simulink model "BloquesLinealizacionRealimentacionNLDesacoplamiento"  (R2023b)
settings: Solver=VariableStepAuto  StartTime=0.0  StopTime=10.0  RelTol=1e-3
values from neighbouring files (symbols this model uses):
  alfa_cu = 3.9E-3    (= 0.0039)    [Parametros.m]
  b_eq = b_m + b_l/(r^2)    (= 2.19444444444e-05)    [Parametros.m]
  C_ts = 0.818    [Parametros.m]
  g = 9.80665    [Parametros.m]
  J_eq = J_m + J_l/(r^2)    [Parametros.m]
  k_l = m*l_cm + m_l(1)*l_l    [Parametros.m]
  L_d = 6.6E-3    (= 0.0066)    [Parametros.m]
  L_ls = 0.8E-3    (= 0.0008)    [Parametros.m]
  L_q = 5.8E-3    (= 0.0058)    [Parametros.m]
  lambda_m = 0.016    [Parametros.m]
  P_p = 3    [Parametros.m]
  r = 120    [Parametros.m]
  R_tsamb = 146.7    [Parametros.m]
  Rs = 1.02    [Parametros.m]
  Tsref = 20    [Parametros.m]
settings Model: Creator=Home  LastModifiedBy=Home

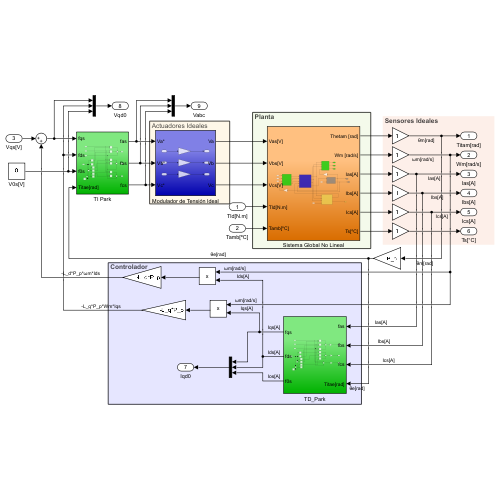
[thumbnail: Simulink's stored preview of the top-level diagram]
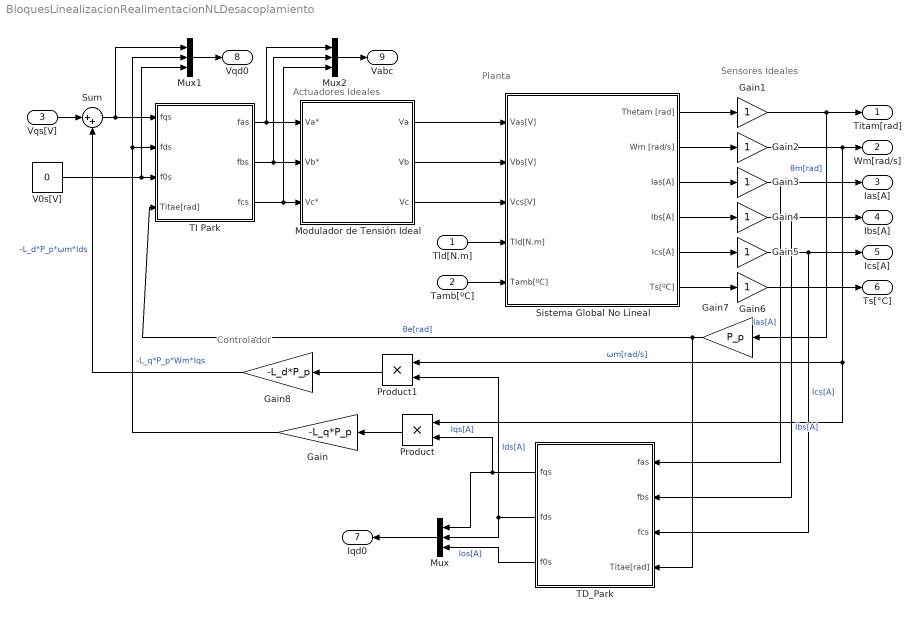
== system BloquesLinealizacionRealimentacionNLDesacoplamiento ==
  note: Planta
  note: Actuadores Ideales
  note: Controlador
  note: Sensores Ideales
  Tld[N.m] : Inport
  Tamb[ºC] : Inport  Port=2
  Vqs[V] : Inport  Port=3
  Gain : Gain  Gain=-L_q*P_p
  Gain{1..6} (6 alike) : Gain
  Gain7 : Gain  Gain=P_p
  Gain8 : Gain  Gain=-L_d*P_p
  Modulador de Tensión Ideal : Subsystem
  Mux : Mux  Inputs=3
  Mux1 : Mux  Inputs=3
  Mux2 : Mux  Inputs=3
  Product : Product
  Product1 : Product
  Sistema Global No Lineal : Subsystem
  Sum : Sum  Inputs=|++
  TD_Park : Subsystem
  TI Park : Subsystem
  V0s[V] : Constant  Value=0
  Titam[rad] : Outport
  Wm[rad/s] : Outport  Port=2
  Ias[A] : Outport  Port=3
  Ibs[A] : Outport  Port=4
  Ics[A] : Outport  Port=5
  Ts[°C] : Outport  Port=6
  Iqd0 : Outport  Port=7
  Vqd0 : Outport  Port=8
  Vabc : Outport  Port=9
  wires:
  Mux2/1 -> Vabc/1
  Sistema Global No Lineal/3(Ias[A]) -> Gain3/1
  Gain5/1 -> TD_Park/3(fcs), Ics[A]/1  "Ics[A]"
  Sistema Global No Lineal/4(Ibs[A]) -> Gain4/1
  Gain2/1 -> Product/1, Product1/1, Wm[rad/s]/1  "ωm[rad/s]"
  TD_Park/1(fqs) -> Mux/1, Product/2  "Iqs[A]"
  Product/1 -> Gain/1
  Tld[N.m]/1 -> Sistema Global No Lineal/4(Tld[N.m])
  TD_Park/2(fds) -> Product1/2, Mux/2  "Ids[A]"
  Gain6/1 -> Ts[°C]/1
  Gain4/1 -> Ibs[A]/1, TD_Park/2(fbs)  "Ibs[A]"
  TI Park/3(fcs) -> Mux2/3, Modulador de Tensión Ideal/3(Vc*)
  Gain3/1 -> TD_Park/1(fas), Ias[A]/1  "Ias[A]"
  Gain/1 -> Mux1/2, TI Park/2(fds)  "-L_q*P_p*Wm*Iqs"
  V0s[V]/1 -> Mux1/3, TI Park/3(f0s)
  Gain7/1 -> TI Park/4(Titae[rad]), TD_Park/4(Titae[rad])  "θe[rad]"
  Sistema Global No Lineal/6(Ts[ºC]) -> Gain6/1
  Sistema Global No Lineal/5(Ics[A]) -> Gain5/1
  Mux/1 -> Iqd0/1
  Modulador de Tensión Ideal/3(Vc) -> Sistema Global No Lineal/3(Vcs[V])
  Sistema Global No Lineal/2(Wm [rad/s]) -> Gain2/1
  Modulador de Tensión Ideal/2(Vb) -> Sistema Global No Lineal/2(Vbs[V])
  Gain1/1 -> Gain7/1, Titam[rad]/1  "θm[rad]"
  TD_Park/3(f0s) -> Mux/3  "Ios[A]"
  Tamb[ºC]/1 -> Sistema Global No Lineal/5(Tamb[ºC])
  TI Park/1(fas) -> Mux2/1, Modulador de Tensión Ideal/1(Va*)
  Sistema Global No Lineal/1(Thetam [rad]) -> Gain1/1
  Modulador de Tensión Ideal/1(Va) -> Sistema Global No Lineal/1(Vas[V])
  TI Park/2(fbs) -> Mux2/2, Modulador de Tensión Ideal/2("Vb* ")
  Mux1/1 -> Vqd0/1
  Product1/1 -> Gain8/1
  Vqs[V]/1 -> Sum/1
  Sum/1 -> Mux1/1, TI Park/1(fqs)
  Gain8/1 -> Sum/2  "-L_d*P_p*ωm*Ids"

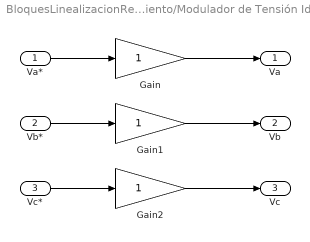
== system BloquesLinealizacionRealimentacionNLDesacoplamiento/Modulador de Tensión Ideal ==
  Va* : Inport
  "Vb* " : Inport  Port=2
  Vc* : Inport  Port=3
  Gain : Gain
  Gain1 : Gain
  Gain2 : Gain
  Va : Outport
  Vb : Outport  Port=2
  Vc : Outport  Port=3
  wires:
  Vc*/1 -> Gain2/1
  "Vb* "/1 -> Gain1/1
  Gain/1 -> Va/1
  Va*/1 -> Gain/1
  Gain1/1 -> Vb/1
  Gain2/1 -> Vc/1

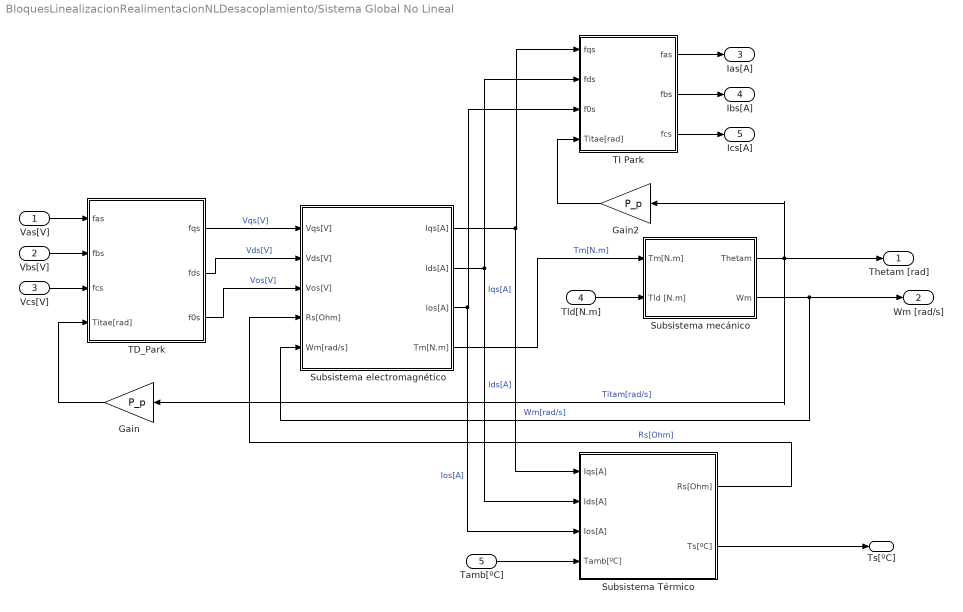
== system BloquesLinealizacionRealimentacionNLDesacoplamiento/Sistema Global No Lineal ==
  Vas[V] : Inport
  Vbs[V] : Inport  Port=2
  Vcs[V] : Inport  Port=3
  Tld[N.m] : Inport  Port=4
  Tamb[ºC] : Inport  Port=5
  Gain : Gain  Gain=P_p
  Gain2 : Gain  Gain=P_p
  Subsistema Térmico : Subsystem
  Subsistema electromagnético : Subsystem
  Subsistema mecánico : Subsystem
  TD_Park : Subsystem
  TI Park : Subsystem
  Thetam [rad] : Outport
  Wm [rad/s] : Outport  Port=2
  Ias[A] : Outport  Port=3
  Ibs[A] : Outport  Port=4
  Ics[A] : Outport  Port=5
  Ts[ºC] : Outport  Port=6
  wires:
  Subsistema electromagnético/3(Ios[A]) -> Subsistema Térmico/3(Ios[A]), TI Park/3(f0s)  "Ios[A]"
  Subsistema mecánico/2(Wm) -> Wm [rad/s]/1, Subsistema electromagnético/5(Wm[rad/s])  "Wm[rad/s]"
  TD_Park/3(f0s) -> Subsistema electromagnético/3(Vos[V])  "Vos[V]"
  Gain/1 -> TD_Park/4(Titae[rad])
  Subsistema Térmico/1(Rs[Ohm]) -> Subsistema electromagnético/4(Rs[Ohm])  "Rs[Ohm]"
  TD_Park/1(fqs) -> Subsistema electromagnético/1(Vqs[V])  "Vqs[V]"
  Vbs[V]/1 -> TD_Park/2(fbs)
  Vcs[V]/1 -> TD_Park/3(fcs)
  Subsistema electromagnético/1(Iqs[A]) -> Subsistema Térmico/1(Iqs[A]), TI Park/1(fqs)  "Iqs[A]"
  Subsistema electromagnético/4(Tm[N.m]) -> Subsistema mecánico/1(Tm[N.m])  "Tm[N.m]"
  Subsistema mecánico/1(Thetam) -> Thetam [rad]/1, Gain2/1, Gain/1  "Titam[rad/s]"
  Tamb[ºC]/1 -> Subsistema Térmico/4(Tamb[ºC])
  Vas[V]/1 -> TD_Park/1(fas)
  TD_Park/2(fds) -> Subsistema electromagnético/2(Vds[V])  "Vds[V]"
  TI Park/2(fbs) -> Ibs[A]/1
  Subsistema electromagnético/2(Ids[A]) -> TI Park/2(fds), Subsistema Térmico/2(Ids[A])  "Ids[A]"
  Gain2/1 -> TI Park/4(Titae[rad])
  TI Park/1(fas) -> Ias[A]/1
  Subsistema Térmico/2(Ts[ºC]) -> Ts[ºC]/1
  Tld[N.m]/1 -> Subsistema mecánico/2(Tld [N.m])
  TI Park/3(fcs) -> Ics[A]/1

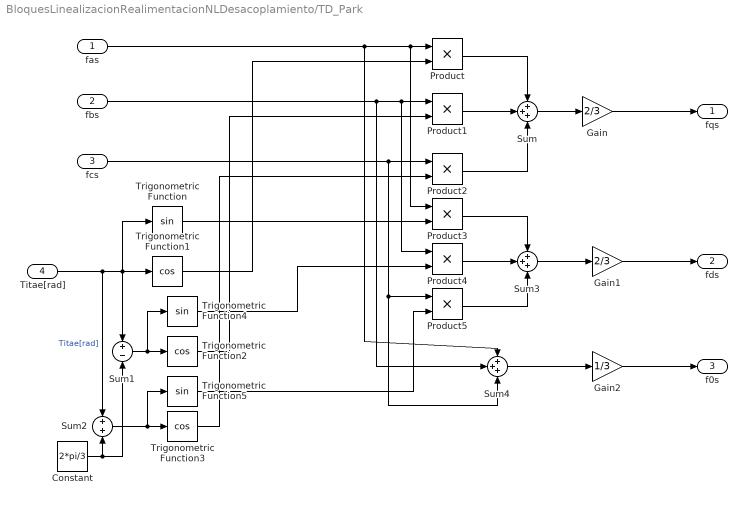
== system BloquesLinealizacionRealimentacionNLDesacoplamiento/TD_Park ==
  fas : Inport
  fbs : Inport  Port=2
  fcs : Inport  Port=3
  Titae[rad] : Inport  Port=4
  Constant : Constant  Value=2*pi/3
  Gain : Gain  Gain=2/3
  Gain1 : Gain  Gain=2/3
  Gain2 : Gain  Gain=1/3
  Product{,1..5} (6 alike) : Product
  Sum : Sum  Inputs=+++
  Sum1 : Sum  Inputs=+-
  Sum2 : Sum
  Sum3 : Sum  Inputs=+++
  Sum4 : Sum  Inputs=+++
  Trigonometric Function : Trigonometry
  Trigonometric Function1 : Trigonometry  Operator=cos
  Trigonometric Function2 : Trigonometry  Operator=cos
  Trigonometric Function3 : Trigonometry  Operator=cos
  Trigonometric Function4 : Trigonometry
  Trigonometric Function5 : Trigonometry
  fqs : Outport
  fds : Outport  Port=2
  f0s : Outport  Port=3
  wires:
  fas/1 -> Sum4/1, Product3/1, Product/1
  Trigonometric Function3/1 -> Product2/2
  Sum1/1 -> Trigonometric Function4/1, Trigonometric Function2/1
  Constant/1 -> Sum2/2, Sum1/2
  Trigonometric Function1/1 -> Product/2
  fcs/1 -> Product5/1, Sum4/3, Product2/1
  Product5/1 -> Sum3/3
  Product/1 -> Sum/1
  Product3/1 -> Sum3/1
  Product1/1 -> Sum/2
  Trigonometric Function/1 -> Product3/2
  Sum2/1 -> Trigonometric Function5/1, Trigonometric Function3/1
  Trigonometric Function5/1 -> Product5/2
  Sum4/1 -> Gain2/1
  fbs/1 -> Sum4/2, Product4/1, Product1/1
  Product2/1 -> Sum/3
  Gain/1 -> fqs/1
  Trigonometric Function4/1 -> Product4/2
  Product4/1 -> Sum3/2
  Trigonometric Function2/1 -> Product1/2
  Gain2/1 -> f0s/1
  Sum/1 -> Gain/1
  Gain1/1 -> fds/1
  Sum3/1 -> Gain1/1
  Titae[rad]/1 -> Sum2/1, Trigonometric Function/1, Sum1/1, Trigonometric Function1/1  "Titae[rad]"

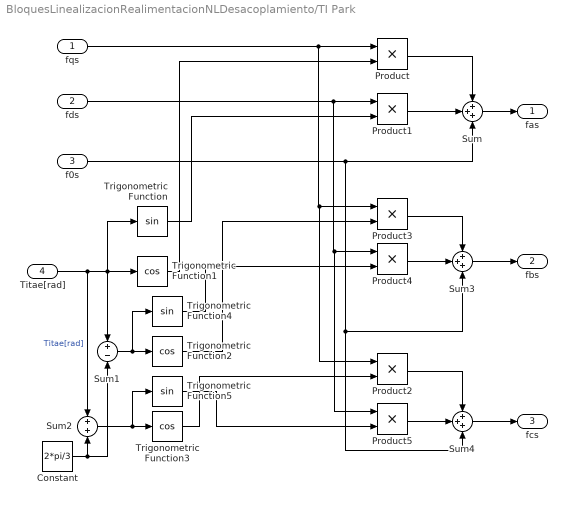
== system BloquesLinealizacionRealimentacionNLDesacoplamiento/TI Park ==
  fqs : Inport
  fds : Inport  Port=2
  f0s : Inport  Port=3
  Titae[rad] : Inport  Port=4
  Constant : Constant  Value=2*pi/3
  Product{,1..5} (6 alike) : Product
  Sum : Sum  Inputs=+++
  Sum1 : Sum  Inputs=+-
  Sum2 : Sum
  Sum3 : Sum  Inputs=+++
  Sum4 : Sum  Inputs=+++
  Trigonometric Function : Trigonometry
  Trigonometric Function1 : Trigonometry  Operator=cos
  Trigonometric Function2 : Trigonometry  Operator=cos
  Trigonometric Function3 : Trigonometry  Operator=cos
  Trigonometric Function4 : Trigonometry
  Trigonometric Function5 : Trigonometry
  fas : Outport
  fbs : Outport  Port=2
  fcs : Outport  Port=3
  wires:
  Constant/1 -> Sum2/2, Sum1/2
  Product1/1 -> Sum/2
  Trigonometric Function2/1 -> Product3/2
  Trigonometric Function5/1 -> Product5/2
  fds/1 -> Product1/1, Product5/1, Product4/1
  f0s/1 -> Sum/3, Sum3/3, Sum4/3
  Product3/1 -> Sum3/1
  fqs/1 -> Product/1, Product2/1, Product3/1
  Product2/1 -> Sum4/1
  Trigonometric Function1/1 -> Product/2
  Product/1 -> Sum/1
  Sum2/1 -> Trigonometric Function5/1, Trigonometric Function3/1
  Sum1/1 -> Trigonometric Function4/1, Trigonometric Function2/1
  Trigonometric Function/1 -> Product1/2
  Product4/1 -> Sum3/2
  Sum/1 -> fas/1
  Trigonometric Function3/1 -> Product2/2
  Product5/1 -> Sum4/2
  Trigonometric Function4/1 -> Product4/2
  Sum3/1 -> fbs/1
  Sum4/1 -> fcs/1
  Titae[rad]/1 -> Sum2/1, Trigonometric Function/1, Sum1/1, Trigonometric Function1/1  "Titae[rad]"

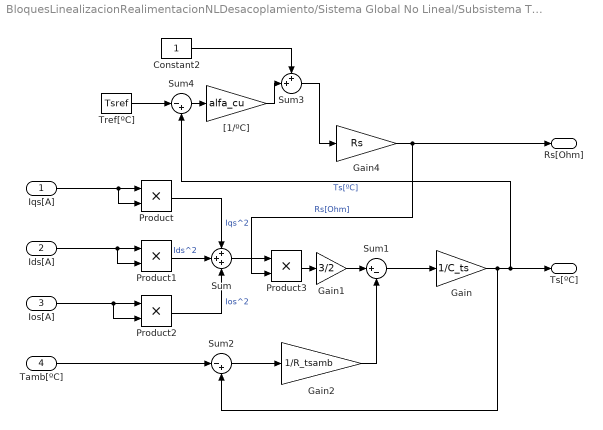
== system BloquesLinealizacionRealimentacionNLDesacoplamiento/Sistema Global No Lineal/Subsistema Térmico ==
  Iqs[A] : Inport
  Ids[A] : Inport  Port=2
  Ios[A] : Inport  Port=3
  Tamb[ºC] : Inport  Port=4
  Constant2 : Constant
  Gain : Gain  Gain=1/C_ts
  Gain1 : Gain  Gain=3/2
  Gain2 : Gain  Gain=1/R_tsamb
  Gain4 : Gain  Gain=Rs
  Product{,1..3} (4 alike) : Product
  Sum : Sum  Inputs=+++
  Sum1 : Sum  Inputs=|+-
  Sum2 : Sum  Inputs=|-+
  Sum3 : Sum  Inputs=++|
  Sum4 : Sum  Inputs=|-+
  Tref[ºC] : Constant  Value=Tsref
  "[1/ºC]" : Gain  Gain=alfa_cu
  Rs[Ohm] : Outport
  Ts[ºC] : Outport  Port=2
  wires:
  Sum3/1 -> Gain4/1
  Gain/1 -> Sum2/2, Ts[ºC]/1, Sum4/2  "Ts[ºC]"
  Product1/1 -> Sum/2  "Ids^2"
  Product/1 -> Sum/1  "Iqs^2"
  Sum/1 -> Product3/1
  Iqs[A]/1 -> Product/2, Product/1
  Ids[A]/1 -> Product1/2, Product1/1
  Product2/1 -> Sum/3  "Ios^2"
  Sum4/1 -> "[1/ºC]"/1
  Tamb[ºC]/1 -> Sum2/1
  Sum1/1 -> Gain/1
  Sum2/1 -> Gain2/1
  Gain4/1 -> Rs[Ohm]/1, Product3/2  "Rs[Ohm]"
  Gain1/1 -> Sum1/1
  Ios[A]/1 -> Product2/2, Product2/1
  Constant2/1 -> Sum3/1
  Tref[ºC]/1 -> Sum4/1
  Product3/1 -> Gain1/1
  "[1/ºC]"/1 -> Sum3/2
  Gain2/1 -> Sum1/2

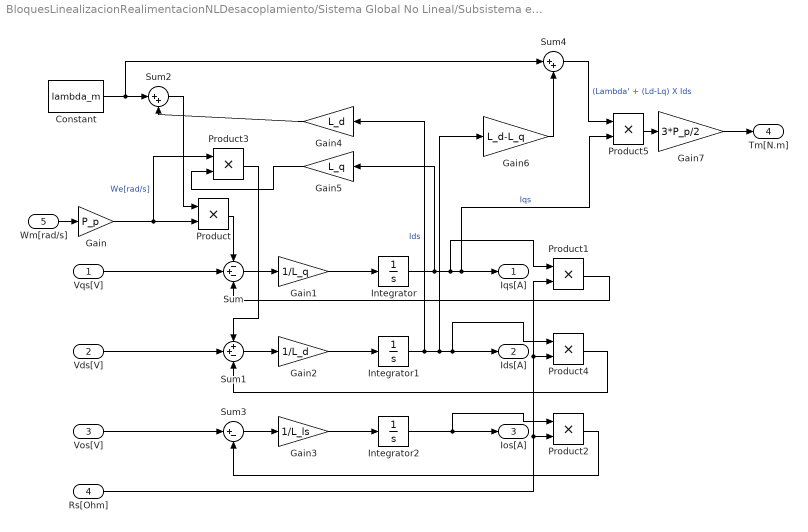
== system BloquesLinealizacionRealimentacionNLDesacoplamiento/Sistema Global No Lineal/Subsistema electromagnético ==
  Vqs[V] : Inport
  Vds[V] : Inport  Port=2
  Vos[V] : Inport  Port=3
  Rs[Ohm] : Inport  Port=4
  Wm[rad/s] : Inport  Port=5
  Constant : Constant  Value=lambda_m
  Gain : Gain  Gain=P_p
  Gain1 : Gain  Gain=1/L_q
  Gain2 : Gain  Gain=1/L_d
  Gain3 : Gain  Gain=1/L_ls
  Gain4 : Gain  Gain=L_d
  Gain5 : Gain  Gain=L_q
  Gain6 : Gain  Gain=L_d-L_q
  Gain7 : Gain  Gain=3*P_p/2
  Integrator : Integrator
  Integrator1 : Integrator
  Integrator2 : Integrator
  Product{,1..5} (6 alike) : Product
  Sum : Sum  Inputs=-+-
  Sum1 : Sum  Inputs=++-
  Sum2 : Sum  Inputs=|++
  Sum3 : Sum  Inputs=|+-
  Sum4 : Sum  Inputs=|++
  Iqs[A] : Outport
  Ids[A] : Outport  Port=2
  Ios[A] : Outport  Port=3
  Tm[N.m] : Outport  Port=4
  wires:
  Product3/1 -> Sum1/1
  Gain5/1 -> Product3/2
  Vos[V]/1 -> Sum3/1
  Sum1/1 -> Gain2/1
  Integrator/1 -> Gain5/1, Product1/1, Iqs[A]/1, Product5/2  "Iqs"
  Integrator2/1 -> Ios[A]/1, Product2/1
  Rs[Ohm]/1 -> Product4/2, Product1/2, Product2/2
  Product1/1 -> Sum/3
  Sum/1 -> Gain1/1
  Sum4/1 -> Product5/1  "(Lambda' + (Ld-Lq) X Ids"
  Integrator1/1 -> Gain6/1, Ids[A]/1, Product4/1, Gain4/1  "Ids"
  Gain/1 -> Product/2, Product3/1  "We[rad/s]"
  Sum3/1 -> Gain3/1
  Gain6/1 -> Sum4/2
  Wm[rad/s]/1 -> Gain/1
  Gain7/1 -> Tm[N.m]/1
  Product5/1 -> Gain7/1
  Vqs[V]/1 -> Sum/2
  Gain2/1 -> Integrator1/1
  Product/1 -> Sum/1
  Constant/1 -> Sum4/1, Sum2/1
  Sum2/1 -> Product/1
  Vds[V]/1 -> Sum1/2
  Gain4/1 -> Sum2/2
  Product4/1 -> Sum1/3
  Product2/1 -> Sum3/2
  Gain1/1 -> Integrator/1
  Gain3/1 -> Integrator2/1

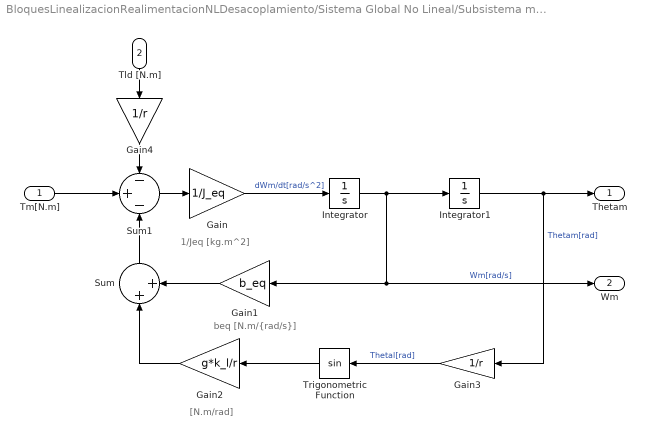
== system BloquesLinealizacionRealimentacionNLDesacoplamiento/Sistema Global No Lineal/Subsistema mecánico ==
  note: beq [N.m/{rad/s}]
  note: 1/Jeq [kg.m^2]
  note: [N.m/rad]
  Tm[N.m] : Inport
  Tld [N.m] : Inport  Port=2
  Gain : Gain  Gain=1/J_eq
  Gain1 : Gain  Gain=b_eq
  Gain2 : Gain  Gain=g*k_l/r
  Gain3 : Gain  Gain=1/r
  Gain4 : Gain  Gain=1/r
  Integrator : Integrator
  Integrator1 : Integrator
  Sum : Sum  Inputs=|++
  Sum1 : Sum  Inputs=-+-
  Trigonometric Function : Trigonometry
  Thetam : Outport
  Wm : Outport  Port=2
  wires:
  Tld [N.m]/1 -> Gain4/1
  Gain3/1 -> Trigonometric Function/1  "Thetal[rad]"
  Gain1/1 -> Sum/2
  Tm[N.m]/1 -> Sum1/2
  Integrator/1 -> Wm/1, Gain1/1, Integrator1/1  "Wm[rad/s]"
  Gain4/1 -> Sum1/1
  Integrator1/1 -> Thetam/1, Gain3/1  "Thetam[rad]"
  Gain2/1 -> Sum/1
  Trigonometric Function/1 -> Gain2/1
  Sum/1 -> Sum1/3
  Gain/1 -> Integrator/1  "dWm/dt[rad/s^2]"
  Sum1/1 -> Gain/1

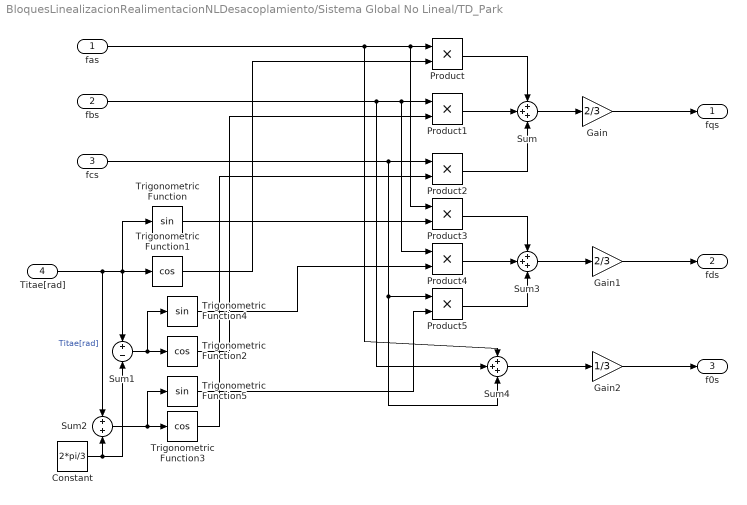
== system BloquesLinealizacionRealimentacionNLDesacoplamiento/Sistema Global No Lineal/TD_Park ==
  fas : Inport
  fbs : Inport  Port=2
  fcs : Inport  Port=3
  Titae[rad] : Inport  Port=4
  Constant : Constant  Value=2*pi/3
  Gain : Gain  Gain=2/3
  Gain1 : Gain  Gain=2/3
  Gain2 : Gain  Gain=1/3
  Product{,1..5} (6 alike) : Product
  Sum : Sum  Inputs=+++
  Sum1 : Sum  Inputs=+-
  Sum2 : Sum
  Sum3 : Sum  Inputs=+++
  Sum4 : Sum  Inputs=+++
  Trigonometric Function : Trigonometry
  Trigonometric Function1 : Trigonometry  Operator=cos
  Trigonometric Function2 : Trigonometry  Operator=cos
  Trigonometric Function3 : Trigonometry  Operator=cos
  Trigonometric Function4 : Trigonometry
  Trigonometric Function5 : Trigonometry
  fqs : Outport
  fds : Outport  Port=2
  f0s : Outport  Port=3
  wires:
  fas/1 -> Sum4/1, Product3/1, Product/1
  Trigonometric Function3/1 -> Product2/2
  Sum1/1 -> Trigonometric Function4/1, Trigonometric Function2/1
  Constant/1 -> Sum2/2, Sum1/2
  Trigonometric Function1/1 -> Product/2
  fcs/1 -> Product5/1, Sum4/3, Product2/1
  Product5/1 -> Sum3/3
  Product/1 -> Sum/1
  Product3/1 -> Sum3/1
  Product1/1 -> Sum/2
  Trigonometric Function/1 -> Product3/2
  Sum2/1 -> Trigonometric Function5/1, Trigonometric Function3/1
  Trigonometric Function5/1 -> Product5/2
  Sum4/1 -> Gain2/1
  fbs/1 -> Sum4/2, Product4/1, Product1/1
  Product2/1 -> Sum/3
  Gain/1 -> fqs/1
  Trigonometric Function4/1 -> Product4/2
  Product4/1 -> Sum3/2
  Trigonometric Function2/1 -> Product1/2
  Gain2/1 -> f0s/1
  Sum/1 -> Gain/1
  Gain1/1 -> fds/1
  Sum3/1 -> Gain1/1
  Titae[rad]/1 -> Sum2/1, Trigonometric Function/1, Sum1/1, Trigonometric Function1/1  "Titae[rad]"

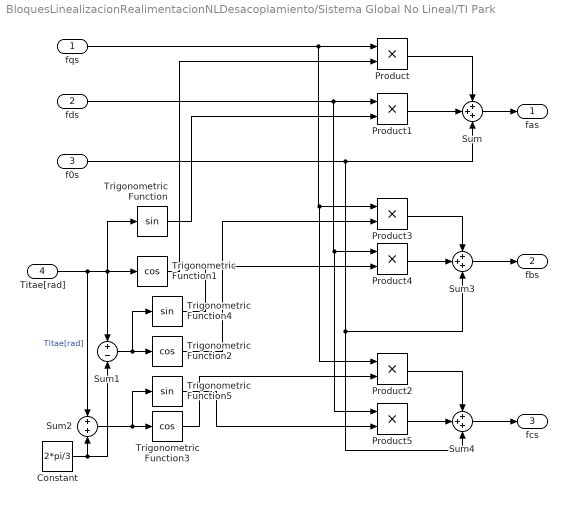
== system BloquesLinealizacionRealimentacionNLDesacoplamiento/Sistema Global No Lineal/TI Park ==
  fqs : Inport
  fds : Inport  Port=2
  f0s : Inport  Port=3
  Titae[rad] : Inport  Port=4
  Constant : Constant  Value=2*pi/3
  Product{,1..5} (6 alike) : Product
  Sum : Sum  Inputs=+++
  Sum1 : Sum  Inputs=+-
  Sum2 : Sum
  Sum3 : Sum  Inputs=+++
  Sum4 : Sum  Inputs=+++
  Trigonometric Function : Trigonometry
  Trigonometric Function1 : Trigonometry  Operator=cos
  Trigonometric Function2 : Trigonometry  Operator=cos
  Trigonometric Function3 : Trigonometry  Operator=cos
  Trigonometric Function4 : Trigonometry
  Trigonometric Function5 : Trigonometry
  fas : Outport
  fbs : Outport  Port=2
  fcs : Outport  Port=3
  wires:
  Constant/1 -> Sum2/2, Sum1/2
  Product1/1 -> Sum/2
  Trigonometric Function2/1 -> Product3/2
  Trigonometric Function5/1 -> Product5/2
  fds/1 -> Product1/1, Product5/1, Product4/1
  f0s/1 -> Sum/3, Sum3/3, Sum4/3
  Product3/1 -> Sum3/1
  fqs/1 -> Product/1, Product2/1, Product3/1
  Product2/1 -> Sum4/1
  Trigonometric Function1/1 -> Product/2
  Product/1 -> Sum/1
  Sum2/1 -> Trigonometric Function5/1, Trigonometric Function3/1
  Sum1/1 -> Trigonometric Function4/1, Trigonometric Function2/1
  Trigonometric Function/1 -> Product1/2
  Product4/1 -> Sum3/2
  Sum/1 -> fas/1
  Trigonometric Function3/1 -> Product2/2
  Product5/1 -> Sum4/2
  Trigonometric Function4/1 -> Product4/2
  Sum3/1 -> fbs/1
  Sum4/1 -> fcs/1
  Titae[rad]/1 -> Sum2/1, Trigonometric Function/1, Sum1/1, Trigonometric Function1/1  "Titae[rad]"
